simulink model "laplace1"  (R2024a)
settings: Solver=VariableStepAuto  StartTime=0.0  StopTime=800  RelTol=1e-3
settings Model: Creator=sabri  LastModifiedBy=sabri

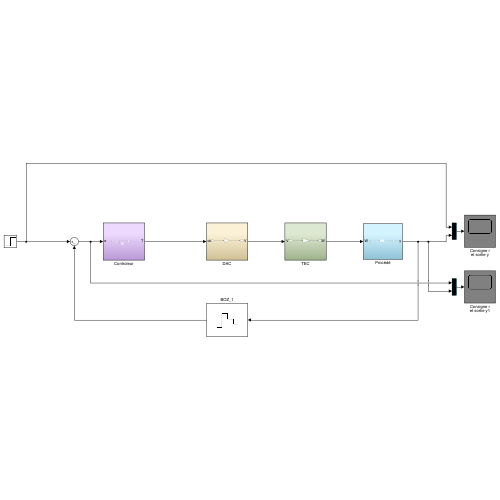
[thumbnail: Simulink's stored preview of the top-level diagram]
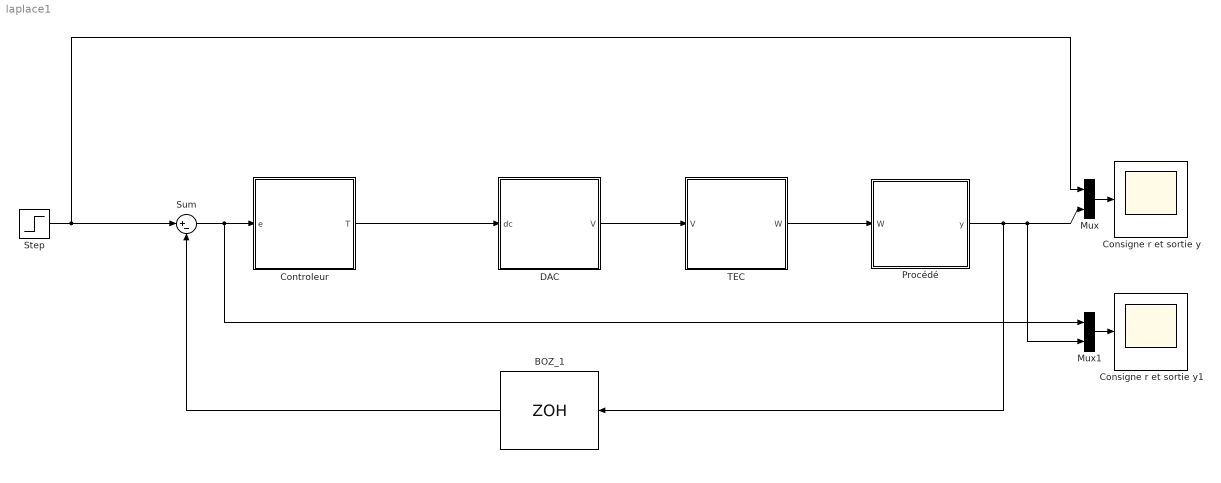
== system laplace1 ==
  BOZ_1 : ZeroOrderHold  SampleTime=0.5
  Consigne r et sortie y : Scope
  Consigne r et sortie y1 : Scope
  Controleur : Subsystem
  DAC : Subsystem
  Mux : Mux  Inputs=2
  Mux1 : Mux  Inputs=2
  Procédé : Subsystem
  Step : Step  Time=10  Before=23  After=28  SampleTime=0
  Sum : Sum  Inputs=|+-
  TEC : Subsystem
  wires:
  Mux/1 -> Consigne r et sortie y/1
  Sum/1 -> Mux1/1, Controleur/1(e)
  Procédé/1(y) -> BOZ_1/1, Mux1/2, Mux/2
  Step/1 -> Mux/1, Sum/1
  TEC/1(W) -> Procédé/1(W)
  Controleur/1(T) -> DAC/1(dc)
  DAC/1(V) -> TEC/1(V)
  Mux1/1 -> Consigne r et sortie y1/1
  BOZ_1/1 -> Sum/2

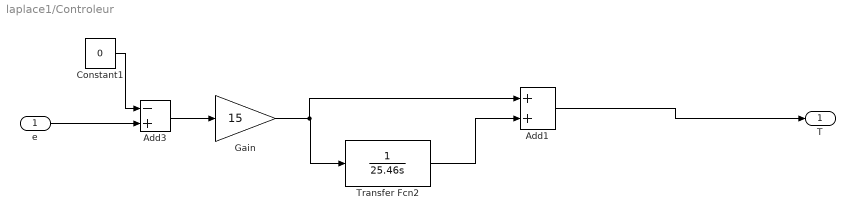
== system laplace1/Controleur ==
  e : Inport
  Add1 : Sum
  Add3 : Sum  Inputs=-+
  Constant1 : Constant  Value=0
  Gain : Gain  Gain=15
  Transfer Fcn2 : TransferFcn  Denominator=[25.46 0]
  T : Outport
  wires:
  e/1 -> Add3/2
  Constant1/1 -> Add3/1
  Add1/1 -> T/1
  Add3/1 -> Gain/1
  Gain/1 -> Add1/1, Transfer Fcn2/1
  Transfer Fcn2/1 -> Add1/2

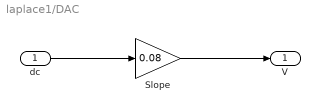
== system laplace1/DAC ==
  dc : Inport
  Slope : Gain  Gain=0.08
  V : Outport
  wires:
  dc/1 -> Slope/1
  Slope/1 -> V/1

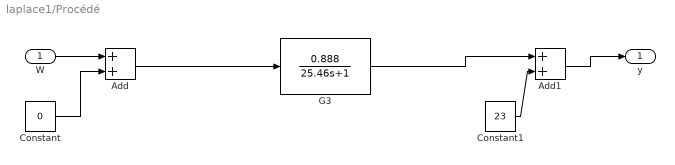
== system laplace1/Procédé ==
  W : Inport
  Add : Sum
  Add1 : Sum
  Constant : Constant  Value=0
  Constant1 : Constant  Value=23
  G3 : TransferFcn  Numerator=[0.888]  Denominator=[25.46 1]
  y : Outport
  wires:
  W/1 -> Add/1
  Constant/1 -> Add/2
  Add1/1 -> y/1
  Constant1/1 -> Add1/2
  G3/1 -> Add1/1
  Add/1 -> G3/1

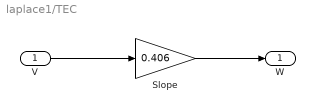
== system laplace1/TEC ==
  V : Inport
  Slope : Gain  Gain=0.406
  W : Outport
  wires:
  Slope/1 -> W/1
  V/1 -> Slope/1
